simulink model "test"  (R2018b)
settings: Solver=VariableStepAuto  StartTime=0.0  StopTime=10.0  RelTol=1e-3
libraries: simulink x1
settings Model: Creator=HP  LastModifiedBy=HP

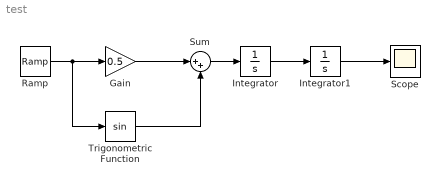
== system test ==
  Gain : Gain  Gain=0.5
  Integrator : Integrator
  Integrator1 : Integrator
  Ramp : simulink/Sources/Ramp  slope=1  start=0  InitialOutput=0
  Scope : Scope
  Sum : Sum  Inputs=|++
  Trigonometric Function : Trigonometry
  wires:
  Ramp/1 -> Trigonometric Function/1, Gain/1
  Gain/1 -> Sum/1
  Trigonometric Function/1 -> Sum/2
  Integrator/1 -> Integrator1/1
  Sum/1 -> Integrator/1
  Integrator1/1 -> Scope/1
